simulink model "SMC_DTC_VS_DTC"  (R2023b)
settings: Solver=FixedStepAuto  StartTime=0.0  StopTime=0.8  FixedStep=0.0000001  MaxStep=0.00001  MinStep=0.0000005
libraries: spsDCVoltageSourceLib x2, spsGroundLib x2, simulink x2, spsThreePhaseVIMeasurementLib x2, spsUniversalBridgeLib x2, sps_lib x1
settings Model: SimulationMode=accelerator  Creator=rainy  LastModifiedBy=rainy
settings SolverCC: ZeroCrossAlgorithm=Adaptive
settings DebuggingCC: MaskedZcDiagnostic=none  IgnoredZcDiagnostic=none

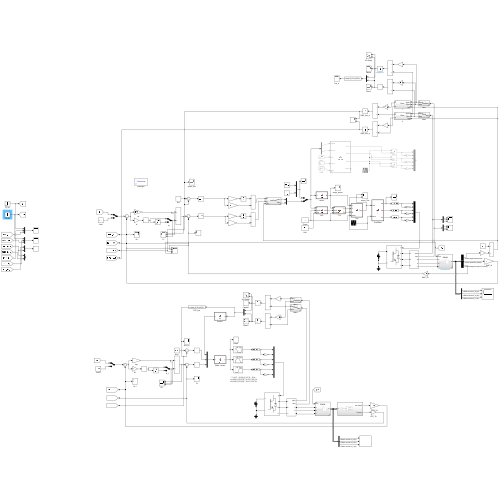
[thumbnail: Simulink's stored preview of the top-level diagram]
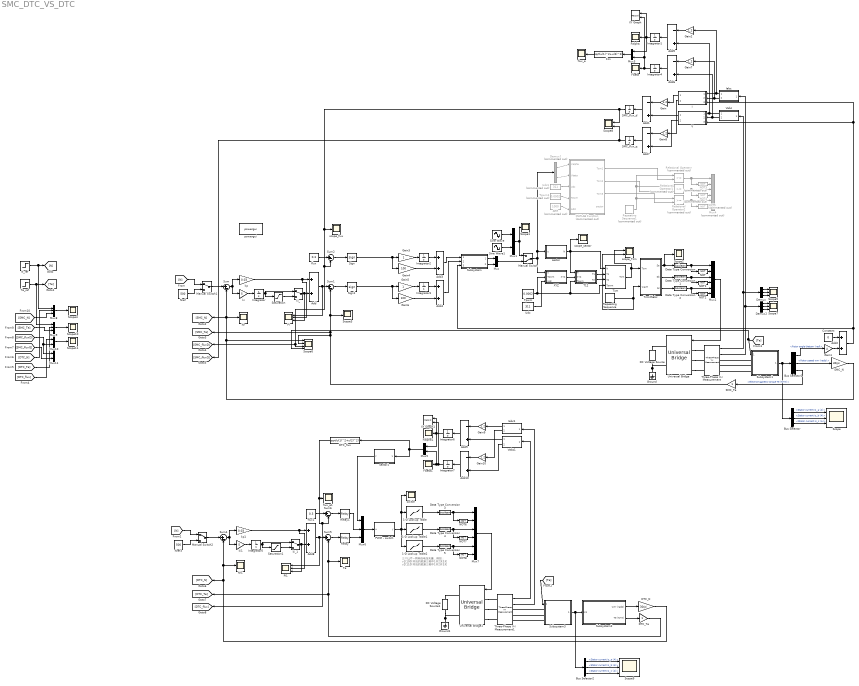
== system SMC_DTC_VS_DTC ==
  note: 三个LUT一同构成电压矢量，例如：
      | v1(100)对应的就是三相中1开2关3关
      | v2(110)对应的就是三相中1开2开3关
  1-D Lookup Table : Lookup_n-D  NumberOfTableDimensions=1  BreakpointsForDimension1=[1 2 3 4 5 6]  Table=[1 1 0 0 0 1]  InternalRulePriority=Speed  RndMeth=Simplest
  1-D Lookup Table1 : Lookup_n-D  NumberOfTableDimensions=1  BreakpointsForDimension1=[1 2 3 4 5 6]  Table=[0 1 1 1 0 0]  InternalRulePriority=Speed  RndMeth=Simplest
  1-D Lookup Table2 : Lookup_n-D  NumberOfTableDimensions=1  BreakpointsForDimension1=[1 2 3 4 5 6]  Table=[0 0 0 1 1 1]  InternalRulePriority=Speed  RndMeth=Simplest
  ARR : Constant  Commented=on  Value=1000
  Add{,2..4,8} (5 alike) : Sum
  Add{1,5..7,9..10} (6 alike) : Sum  Inputs=-+
  Bus Selector : BusSelector  OutputSignals=Stator current is_a (A),Stator current is_b (A),Stator current is_c (A)
  Bus Selector1 : BusSelector  OutputSignals=Rotor angle thetam (rad),Rotor speed wm (rad/s),Electromagnetic torque Te (N*m)
  Bus Selector2 : BusSelector  OutputSignals=Stator current is_a (A),Stator current is_b (A),Stator current is_c (A)
  Constant : Constant  Value=0
  DC Voltage Source : spsDCVoltageSourceLib/DC Voltage Source  Amplitude=311  Measurements=Voltage
  DC Voltage Source1 : spsDCVoltageSourceLib/DC Voltage Source  Amplitude=311  Measurements=Voltage
  DTC_N : Gain  Gain=30/pi
  DTC_Te : Gain
  DTC_flux : Fcn  Expr=sqrt(u(1)^2+u(2)^2)
  Data Type Conversion{,1..5} (6 alike) : DataTypeConversion  OutDataTypeStr=boolean  SaturateOnIntegerOverflow=off  RndMeth=Floor
  Demux : Demux  Outputs=3
  Demux1 : Demux  Commented=on  Outputs=2
  Demux2 : Demux  Outputs=3
  Falpha : Scope
  Falpha1 : Scope
  Fbeta : Scope
  Fbeta1 : Scope
  Fcn : Fcn  Expr=sqrt(u(1)^2+u(2)^2)
  Gain{,2,7..10} (6 alike) : Gain  Gain=1.2
  Gain1 : Gain  Gain=4
  Gain3 : Gain
  Gain4 : Gain  Gain=100
  Gain5 : Gain
  Gain6 : Gain  Gain=100
  Ground : spsGroundLib/Ground  LConnTagsString=a
  Ground1 : spsGroundLib/Ground  LConnTagsString=a
  I : Subsystem  ReferencedSubsystem=Park
  Iabc : Subsystem  ReferencedSubsystem=Clark
  Iabc1 : Subsystem  ReferencedSubsystem=Clark
  Integrator{,1..7} (8 alike) : Integrator
  MATLAB Function : MATLAB Function  Commented=on  TreatAsAtomicUnit=on
  Manual Switch : ManualSwitch  CurrentSetting=0
  Manual Switch1 : ManualSwitch
  Manual Switch2 : ManualSwitch
  Mux{,1,3,5,10..11} (6 alike) : Mux  Inputs=2
  Mux2 : Mux  Inputs=6
  Mux4 : Mux  Commented=on  Inputs=6
  Mux6 : Mux  Inputs=3
  Mux7 : Mux  Inputs=6
  Mux8 : Mux  Inputs=3
  Mux9 : Mux  Inputs=3
  NOT{,1..2,6..8} (6 alike) : Logic  Operator=NOT  IconShape=distinctive  AllPortsSameDT=off  OutDataTypeStr=boolean
  NOT3 : Logic  Commented=on  Operator=NOT  IconShape=distinctive  AllPortsSameDT=off  OutDataTypeStr=boolean
  NOT4 : Logic  Commented=on  Operator=NOT  IconShape=distinctive  AllPortsSameDT=off  OutDataTypeStr=boolean
  NOT5 : Logic  Commented=on  Operator=NOT  IconShape=distinctive  AllPortsSameDT=off  OutDataTypeStr=boolean
  N_ref : Step  Time=0.4  Before=200  After=400  SampleTime=0
  Nr : Scope
  Nr1 : Scope
  Nref : Constant  Value=500
  Nref3 : Constant  Value=500
  PI : Scope  NumInputPorts=3
  PI1 : Scope  NumInputPorts=3
  PWM - switch : MATLAB Function  TreatAsAtomicUnit=on
  Relational Operator : RelationalOperator  Commented=on  OutDataTypeStr=boolean  RndMeth=Simplest  InputSameDT=off
  Relational Operator1 : RelationalOperator  Commented=on  OutDataTypeStr=boolean  RndMeth=Simplest  InputSameDT=off
  Relational Operator2 : RelationalOperator  Commented=on  OutDataTypeStr=boolean  RndMeth=Simplest  InputSameDT=off
  Relay : Relay  OnSwitchValue=0.1  OffSwitchValue=-0.1
  Relay1 : Relay  OnSwitchValue=0.002  OffSwitchValue=-0.002
  Repeating Sequence : simulink/Sources/Repeating Sequence  rep_seq_t=[0 0.0001 0.0002]  rep_seq_y=[0 10 0]
  Repeating Sequence1 : simulink/Sources/Repeating Sequence  Commented=on  rep_seq_t=[0 0.0001 0.0002]  rep_seq_y=[0 1000 0]
  SMC_N : Gain  Gain=30/pi
  SMC_Te : Gain
  SMC_flux_d : Integrator
  SMC_flux_q : Integrator
  Saturation : Saturate  UpperLimit=10  LowerLimit=-10  ZeroCross=off
  Saturation1 : Saturate  UpperLimit=10  LowerLimit=-10
  Scope{,5,7,9} (4 alike) : Scope  NumInputPorts=3
  Scope{1..4,10..11} (6 alike) : Scope
  Scope6 : Scope  NumInputPorts=4
  Scope8 : Scope  NumInputPorts=2
  Sign : Signum
  Sign1 : Signum
  Sine Wave : Sin  Amplitude=200  Frequency=50*pi  Phase=-pi/2  SampleTime=0
  Sine Wave1 : Sin  Amplitude=200  Frequency=50*pi  SampleTime=0
  Subsystem : Subsystem  ReferencedSubsystem=AntiPark
  Subsystem1 : Subsystem  ReferencedSubsystem=PMSM
  Subsystem2 : Subsystem
  Subsystem3 : Subsystem  ReferencedSubsystem=PMSM
  Sum{,1..2,4..6} (6 alike) : Sum  Inputs=|+-
  T12 : MATLAB Function  TreatAsAtomicUnit=on
  Tcm : MATLAB Function  TreatAsAtomicUnit=on
  Tcm2Sabc : MATLAB Function  TreatAsAtomicUnit=on
  Te : Scope
  Te_ref : Step  Time=0.2  After=3  SampleTime=0
  Three-Phase V-I Measurement : spsThreePhaseVIMeasurementLib/Three-Phase V-I Measurement  VoltageMeasurement=phase-to-ground  SetLabelV=off  LabelV=Vabc  Vpu=off  VpuLL=off  CurrentMeasurement=yes  SetLabelI=off  LabelI=Iabc  Ipu=off  Pbase=100e6  Vbase=500e3  OutputType=Complex  PhasorSimulation=off  PSBequivalent=0
  Three-Phase V-I Measurement1 : spsThreePhaseVIMeasurementLib/Three-Phase V-I Measurement  VoltageMeasurement=phase-to-ground  SetLabelV=off  LabelV=Vabc  Vpu=off  VpuLL=off  CurrentMeasurement=yes  SetLabelI=off  LabelI=Iabc  Ipu=off  Pbase=100e6  Vbase=500e3  OutputType=Complex  PhasorSimulation=off  PSBequivalent=0
  Tpwm : Constant  Value=0.0002
  Tpwm1 : Constant  Commented=on  Value=0.0002
  Udc : Constant  Value=311
  Udc1 : Constant  Commented=on  Value=311
  Universal Bridge : spsUniversalBridgeLib/Universal Bridge  Arms=3  SnubberResistance=1e5  SnubberCapacitance=inf  Device=IGBT / Diodes  Ron=1e-3  Lon=0  ForwardVoltages="[  0  0  ]"  ForwardVoltage=0  GTOparameters=[ 10e-6 , 20e-6 ]  IGBTparameters=[ 1e-6 , 2e-6 ]  Measurements=None  Measurements_2=None  converterType=Rectifier
  Universal Bridge1 : spsUniversalBridgeLib/Universal Bridge  Arms=3  SnubberResistance=1e5  SnubberCapacitance=inf  Device=IGBT / Diodes  Ron=1e-3  Lon=0  ForwardVoltages="[  0  0  ]"  ForwardVoltage=0  GTOparameters=[ 10e-6 , 20e-6 ]  IGBTparameters=[ 1e-6 , 2e-6 ]  Measurements=None  Measurements_2=None  converterType=Rectifier
  V : Subsystem  ReferencedSubsystem=Park
  Vabc : Subsystem  ReferencedSubsystem=Clark
  Vabc1 : Subsystem  ReferencedSubsystem=Clark
  XY Graph : Record  FileSettingsInternal="{\"entries\":[{\"content\":{\"excelSettings\":{\"content\":{},\"type\":\"Streamout.ExcelSettings\"}},\"type\":\"Streamout.FileSettingStorage\",\"uuid\":\"\"}],\"packageUris\":[\"http:\\/\\/schema.mathworks.com\\/mf0\\/streamout_blocks\\/R2020a\"],\"version\":\"1.0\"}"  Layout=[1 1]  SignalsInternal="{\"entries\":[{\"content\":{\"signals\":[{\"content\":{\"blockPath\":[],\"dimensions\":[1],\"domain\":\"\",\"lineColor\":\"#64d413\",\"plots\":[1],\"port\":1,\"sid\":[\"\"],\"signalID\":32394,\"signalName\":\"Integrator1\"},\"type\":\"RecordBlkView.Signal\",\"uuid\":\"\"},{\"content\":{\"blockPath\":[],\"dimensions\":[1],\"domain\":\"\",\"lineColor\":\"#ff13a6\",\"plots\":[1],\"port\":2,\"sid\":[\"\"],\"signalID\":32398,\"signalName\":\"Integrator4\"},\"type\":\"RecordBlkView.Signal\",\"uuid\":\"\"}]},\"type\":\"RecordBlkView.InputSignals\",\"uuid\":\"\"}],\"packageUris\":[\"http:\\/\\/schema.mathworks.com\\/mf0\\/streamout_blocks\\/R2020a\"],\"version\":\"1.0\"}"  VisualizationBindings="{\"xyplotplugin\":{\"info\":[{\"series\":[{\"bindingParametersList\":[{\"parameter\":\"X-Axis\",\"signalID\":32394,\"signalName\":\"Integrator1\"},{\"parameter\":\"Y-Axis\",\"signalID\":32398,\"signalName\":\"Integrator4\"}],\"seriesID\":40381}],\"subplotID\":1}]}}"  CompatibilityTag=XY  st=-1
  XY Graph1 : Record  FileSettingsInternal="{\"entries\":[{\"content\":{\"excelSettings\":{\"content\":{},\"type\":\"Streamout.ExcelSettings\"}},\"type\":\"Streamout.FileSettingStorage\",\"uuid\":\"\"}],\"packageUris\":[\"http:\\/\\/schema.mathworks.com\\/mf0\\/streamout_blocks\\/R2020a\"],\"version\":\"1.0\"}"  Layout=[1 1]  SignalsInternal="{\"entries\":[{\"content\":{\"signals\":[{\"content\":{\"blockPath\":[],\"dimensions\":[1],\"domain\":\"\",\"lineColor\":\"#a2142f\",\"plots\":[1],\"port\":1,\"sid\":[\"\"],\"signalID\":32402,\"signalName\":\"Integrator6\"},\"type\":\"RecordBlkView.Signal\",\"uuid\":\"\"},{\"content\":{\"blockPath\":[],\"dimensions\":[1],\"domain\":\"\",\"lineColor\":\"#139fff\",\"plots\":[1],\"port\":2,\"sid\":[\"\"],\"signalID\":32406,\"signalName\":\"Integrator7\"},\"type\":\"RecordBlkView.Signal\",\"uuid\":\"\"}]},\"type\":\"RecordBlkView.InputSignals\",\"uuid\":\"\"}],\"packageUris\":[\"http:\\/\\/schema.mathworks.com\\/mf0\\/streamout_blocks\\/R2020a\"],\"version\":\"1.0\"}"  VisualizationBindings="{\"xyplotplugin\":{\"info\":[{\"series\":[{\"bindingParametersList\":[{\"parameter\":\"X-Axis\",\"signalID\":32402,\"signalName\":\"Integrator6\"},{\"parameter\":\"Y-Axis\",\"signalID\":32406,\"signalName\":\"Integrator7\"}],\"seriesID\":47759}],\"subplotID\":1}]}}"  CompatibilityTag=XY  st=-1
  XYZ : MATLAB Function  TreatAsAtomicUnit=on
  flux : Constant  Value=0.3
  flux1 : Constant  Value=0.3
  flux_a : Scope
  flux_a1 : Scope
  ki : Gain  Gain=5
  ki1 : Gain  Gain=5
  ki_ : ManualSwitch
  ki_1 : ManualSwitch
  kp : Gain  Gain=0.03
  kp1 : Gain  Gain=0.03
  powergui : sps_lib/powergui  Priority=1  SimulationMode=Continuous  SampleTime=50e-6  frequency=60  Iterations=50  frequencyindice=0  Pbase=100e6  ErrMax=1e-4  UnitsV=kV  UnitsW=MW  buscounter=0  FunctionMessages=off  echomessages=off  EnableUseOfTLC=off  CurrentSourceSwitches=off  DisableSnubberDevices=off  DisableRonSwitches=off  DisableVfSwitches=off  DisplayEquations=off  AutomaticDiscreteSolvers=off  SolverType=Tustin/Backward Euler (TBE)  Interpol=off  ExternalGateDelay=off  methode=off  Ts=100  x0status=blocks  SPID=on  SwTol=0  HookPort=off  NonlinearTolerance=1e-4  nMaxIteration=100  ContinueOnMaxIteration=off  RestoreLinks=warning  ResistiveCurrentMeasurement=off  Frange=[0:2:500]  Ylog=off  Xlog=on  ShowGrid=off  save=off  variable=ZData  structure=0  ZoomFFT=off  StartTime=0.0  cycles=1  DisplayStyle=1  fundamental=60  FreqAxis=off  MaxFrequency=1000  frequencyindicesteady=1  RmsSteady=1  display=off
  scope_Tcm : Scope  NumInputPorts=2
  scope_flux : Scope
  scope_sector : Scope
  sector : MATLAB Function  TreatAsAtomicUnit=on
  sector1 : MATLAB Function  TreatAsAtomicUnit=on
  switch : Scope
  wires:
  [Te] -> Scope6/4, Subsystem1/1
  Bus Selector/2 -> Scope/2  "<Stator current is_b (A)>"
  Bus Selector/3 -> Scope/3  "<Stator current is_c (A)>"
  Bus Selector/1 -> Scope/1  "<Stator current is_a (A)>"
  Bus Selector1/2 -> SMC_N/1  "<Rotor speed wm (rad/s)>"
  Bus Selector1/3 -> SMC_Te/1  "<Electromagnetic torque Te (N*m)>"
  ki_/1 -> PI/3, Add/2
  Saturation/1 -> ki_/2
  SMC_N/1 -> Scope6/1, Sum/2, [SMC_N], Nr/1
  kp/1 -> PI/2, Add/1
  Integrator/1 -> ki_/1, Saturation/1
  ki/1 -> Integrator/1
  Add/1 -> Sum1/1, PI/1
  Sum/1 -> ki/1, kp/1
  Nref/1 -> Manual Switch1/2
  Add1/1 -> SMC_flux_d/1
  Three-Phase V-I Measurement/2 -> Demux2/1, Iabc/1
  Gain/1 -> Add1/1
  Three-Phase V-I Measurement/1 -> Demux/1, Vabc/1
  Iabc/1 -> Gain2/1, I/1
  Iabc/2 -> Gain7/1, I/2
  I/1 -> Gain/1
  Vabc/1 -> Add5/2, V/1
  Vabc/2 -> V/2, Add6/2
  V/1 -> Add1/2
  flux/1 -> Sum2/1
  SMC_flux_d/1 -> Scope8/1, Scope6/3, [SMC_fluxD], Sum2/2, scope_flux/1
  Gain1/1 -> Add2/2
  Constant/1 -> Add2/1
  Bus Selector1/1 -> Gain1/1  "<Rotor angle thetam (rad)>"
  Tpwm/1 -> Tcm/4(Tpwm), T12/3(Tpwm), XYZ/2(Tpwm)
  Udc/1 -> XYZ/3(Udc)
  XYZ/1(XYZ) -> T12/2(XYZ)
  sector/1(N) -> scope_sector/1, Tcm/1(N), T12/1(N)
  T12/1(T1) -> Tcm/2(T1)
  T12/2(T2) -> Tcm/3(T2)
  Tcm/1(Tcm) -> scope_Tcm/1, Tcm2Sabc/1(Tcm)
  Repeating Sequence/1 -> Tcm2Sabc/2(wave), scope_Tcm/2
  NOT/1 -> Mux2/2
  Tcm2Sabc/3(Sc) -> Data Type Conversion2/1
  Data Type Conversion1/1 -> NOT1/1, Mux2/3
  Data Type Conversion2/1 -> NOT2/1, Mux2/5
  Tcm2Sabc/2(Sb) -> Data Type Conversion1/1
  Tcm2Sabc/1(Sa) -> Scope2/1, Data Type Conversion/1
  NOT1/1 -> Mux2/4
  Data Type Conversion/1 -> NOT/1, Mux2/1
  NOT2/1 -> Mux2/6
  Subsystem/1 -> Mux/1
  Subsystem/2 -> Mux/2
  Manual Switch/1 -> XYZ/1(u), Demux1/1, sector/1(u)
  Mux/1 -> Manual Switch/2
  Mux1/1 -> Scope1/1, Manual Switch/1
  Sine Wave/1 -> Mux1/1
  Sine Wave1/1 -> Mux1/2
  Sign/1 -> Gain4/1, Gain3/1
  Gain3/1 -> Integrator2/1
  Integrator2/1 -> Add3/1
  Gain4/1 -> Add3/2
  Sign1/1 -> Gain6/1, Gain5/1
  Gain6/1 -> Add4/2
  Integrator3/1 -> Add4/1
  Gain5/1 -> Integrator3/1
  Sum1/1 -> Sign1/1
  Sum2/1 -> Sign/1
  Add4/1 -> Subsystem/2
  Subsystem1/1 -> Bus Selector1/1, Bus Selector/1
  Demux/1 -> Scope5/1
  Demux/2 -> Scope5/2
  Demux/3 -> Scope5/3
  Demux1/1 -> MATLAB Function/1(Valpha)
  Demux1/2 -> MATLAB Function/2(Vbeta)
  Udc1/1 -> MATLAB Function/3(Udc)
  Tpwm1/1 -> MATLAB Function/4(Tpwm)
  ARR/1 -> MATLAB Function/5(ARR)
  MATLAB Function/3(Tcm3) -> Relational Operator2/2
  Relational Operator2/1 -> NOT5/1, Mux4/5
  NOT3/1 -> Mux4/2
  NOT5/1 -> Mux4/6
  Relational Operator1/1 -> NOT4/1, Mux4/3
  Relational Operator/1 -> NOT3/1, Mux4/1
  NOT4/1 -> Mux4/4
  MATLAB Function/2(Tcm2) -> Relational Operator1/2
  Repeating Sequence1/1 -> Relational Operator2/1, Relational Operator1/1, Relational Operator/1
  MATLAB Function/1(Tcm1) -> Relational Operator/2
  Mux2/1 -> Universal Bridge/1
  Add2/1 -> I/3, V/3, Subsystem/3
  Integrator1/1 -> Mux3/1, Falpha/1, XY Graph/1
  Integrator4/1 -> Mux3/2, XY Graph/2, Fbeta/1
  Gain2/1 -> Add5/1
  Add5/1 -> Integrator1/1
  Gain7/1 -> Add6/1
  Add6/1 -> Integrator4/1
  Fcn/1 -> flux_a/1
  Mux3/1 -> Fcn/1
  V/2 -> Add7/2
  Add7/1 -> SMC_flux_q/1
  I/2 -> Gain8/1
  Gain8/1 -> Add7/1
  SMC_flux_q/1 -> [SMC_fluxQ], Scope8/2
  Demux2/3 -> Scope7/3
  Demux2/2 -> Scope7/2
  Demux2/1 -> Scope7/1
  Add3/1 -> Subsystem/1
  Manual Switch1/1 -> Sum/1
  [N] -> Manual Switch1/1
  Integrator7/1 -> XY Graph1/2, Mux5/2, Fbeta1/1
  Add8/1 -> PI1/1, Sum5/1
  Data Type Conversion4/1 -> Mux7/3, NOT7/1
  Iabc1/2 -> Gain10/1
  Mux5/1 -> sector1/1(u), DTC_flux/1
  Add10/1 -> Integrator7/1
  Vabc1/2 -> Add10/2
  Integrator6/1 -> XY Graph1/1, Mux5/1, Falpha1/1
  Bus Selector2/2 -> Scope9/2  "<Stator current is_b (A)>"
  Relay/1 -> Mux6/3
  NOT7/1 -> Mux7/4
  Three-Phase V-I Measurement1/2 -> Iabc1/1
  Subsystem3/1 -> Bus Selector2/1, Subsystem2/1(In1)
  ki_1/1 -> PI1/3, Add8/2
  1-D Lookup Table1/1 -> Data Type Conversion4/1
  NOT6/1 -> Mux7/2
  Integrator5/1 -> ki_1/1, Saturation1/1
  sector1/1(y) -> Mux6/1
  Relay1/1 -> Mux6/2
  Mux7/1 -> Universal Bridge1/1
  1-D Lookup Table2/1 -> Data Type Conversion5/1
  PWM - switch/1(y) -> 1-D Lookup Table2/1, switch/1, 1-D Lookup Table/1, 1-D Lookup Table1/1
  Saturation1/1 -> ki_1/2
  1-D Lookup Table/1 -> Data Type Conversion3/1
  Manual Switch2/1 -> Sum4/1
  Data Type Conversion3/1 -> NOT6/1, Mux7/1
  Gain10/1 -> Add10/1
  Mux6/1 -> PWM - switch/1(u)
  Bus Selector2/1 -> Scope9/1  "<Stator current is_a (A)>"
  DTC_flux/1 -> Sum6/2, [DTC_flux], flux_a1/1
  Sum5/1 -> Relay/1
  Vabc1/1 -> Add9/2
  Data Type Conversion5/1 -> Mux7/5, NOT8/1
  Subsystem2/2(Te (N*m)) -> DTC_Te/1
  DTC_N/1 -> [DTC_N], Sum4/2, Nr1/1
  Subsystem2/1(wm (rad/s)) -> DTC_N/1
  kp1/1 -> PI1/2, Add8/1
  Add9/1 -> Integrator6/1
  Bus Selector2/3 -> Scope9/3  "<Stator current is_c (A)>"
  Iabc1/1 -> Gain9/1
  Sum6/1 -> Relay1/1
  Sum4/1 -> ki1/1, kp1/1
  flux1/1 -> Sum6/1
  Gain9/1 -> Add9/1
  Three-Phase V-I Measurement1/1 -> Vabc1/1
  ki1/1 -> Integrator5/1
  NOT8/1 -> Mux7/6
  N_ref/1 -> Mux8/1, [N]
  [N] -> Manual Switch2/1
  Nref3/1 -> Manual Switch2/2
  [Te] -> Subsystem3/1
  Te_ref/1 -> Mux9/1, [Te]
  DTC_Te/1 -> [DTC_Te], Te/1, Sum5/2
  SMC_Te/1 -> [SMC_Te], Sum1/2, Scope3/1, Scope6/2
  [SMC_N] -> Mux8/3
  [DTC_N] -> Mux8/2
  [SMC_Te] -> Mux9/3
  [DTC_Te] -> Mux9/2
  [SMC_fluxD] -> Mux10/2, Mux11/1
  [DTC_flux] -> Mux10/1
  [SMC_fluxQ] -> Mux11/2
  Mux8/1 -> Scope4/1
  Mux9/1 -> Scope10/1
  Mux10/1 -> Scope11/1
  connections:
  Ground/LConn1 -- Universal Bridge/RConn2 -- DC Voltage Source/LConn1
  Universal Bridge/LConn3 -- Three-Phase V-I Measurement/LConn3
  Subsystem1/LConn3 -- Three-Phase V-I Measurement/RConn3
  Subsystem1/LConn1 -- Three-Phase V-I Measurement/RConn1
  Universal Bridge/LConn2 -- Three-Phase V-I Measurement/LConn2
  Subsystem1/LConn2 -- Three-Phase V-I Measurement/RConn2
  Universal Bridge/LConn1 -- Three-Phase V-I Measurement/LConn1
  DC Voltage Source/RConn1 -- Universal Bridge/RConn1
  Ground1/LConn1 -- Universal Bridge1/RConn2 -- DC Voltage Source1/LConn1
  Subsystem3/LConn3 -- Three-Phase V-I Measurement1/RConn3
  Subsystem3/LConn1 -- Three-Phase V-I Measurement1/RConn1
  Subsystem3/LConn2 -- Three-Phase V-I Measurement1/RConn2
  Universal Bridge1/LConn2 -- Three-Phase V-I Measurement1/LConn2
  Universal Bridge1/LConn1 -- Three-Phase V-I Measurement1/LConn1
  Universal Bridge1/LConn3 -- Three-Phase V-I Measurement1/LConn3
  DC Voltage Source1/RConn1 -- Universal Bridge1/RConn1

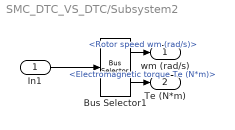
== system SMC_DTC_VS_DTC/Subsystem2 ==
  In1 : Inport
  Bus Selector1 : BusSelector  OutputSignals=Rotor speed wm (rad/s),Electromagnetic torque Te (N*m)
  wm (rad/s) : Outport
  Te (N*m) : Outport  Port=2
  wires:
  Bus Selector1/2 -> Te (N*m)/1  "<Electromagnetic torque Te (N*m)>"
  Bus Selector1/1 -> wm (rad/s)/1  "<Rotor speed wm (rad/s)>"
  In1/1 -> Bus Selector1/1

== matlab function SMC_DTC_VS_DTC/XYZ ==
  data: u input; XYZ output; Tpwm input; Udc input
function XYZ = fcn(u, Tpwm, Udc)

XYZ = zeros([1 3]);
XYZ(1) = Tpwm/Udc * sqrt(3)*u(2);
XYZ(2) = Tpwm/Udc * (3/2*u(1) + sqrt(3)/2*u(2));
XYZ(3) = Tpwm/Udc * (-3/2*u(1) + sqrt(3)/2*u(2));

== matlab function SMC_DTC_VS_DTC/sector ==
  data: u input; N output
function N = fcn(u)

if(u(1) == 0)
    i = 4;
else
    % 将\psi_{\aplha}和\psi_{\beta}分解为三相
    a1 = u(2);
    b1 = u(2)*(-0.5) + sqrt(3)/2*u(1);
    c1 = u(2)*(-0.5) - sqrt(3)/2*u(1);

    if(a1 > 0)
        a = 1;
    else
        a = 0;
    end
    
    if(b1 > 0)
        b = 1;
    else
        b = 0;
    end
    
    if(c1 > 0)
        c = 1;
    else
        c = 0;
    end

    % i = 4*a+2*b+c;
    i = 4*c+2*b+a;
end

% Sector_table=[4 6 5 2 3 1];
% 
% N = Sector_table(i);
N = i;

== matlab function SMC_DTC_VS_DTC/T12 ==
  data: N input; XYZ input; T1 output; Tpwm input; T2 output
function [T1, T2] = fcn(N, XYZ, Tpwm)

X = XYZ(1);
Y = XYZ(2);
Z = XYZ(3);

switch (N)
    case 1
        T1 = Z; T2 = Y;
    case 2
        T1 = Y; T2 = -X;
    case 3
        T1 = -Z; T2 = X;
    case 4
        T1 = -X; T2 = Z;
    case 5
        T1 = X; T2 = -Y;
    otherwise
        T1 = -Y; T2 = -Z;
end

if T1 + T2 > Tpwm
    T1 = T1/(T1 + T2)*Tpwm;
    T2 = T2/(T1 + T2)*Tpwm;
end

== matlab function SMC_DTC_VS_DTC/Tcm ==
  data: N input; T1 input; T2 input; Tcm output; Tpwm input
function Tcm = fcn(N, T1, T2, Tpwm)

Tcm = zeros([1 3]);

Ta = (Tpwm - T1 - T2)/4;
Tb = Ta + T1/2;
Tc = Tb + T2/2;

switch(N)
    case 1
        Tcm(1) = Tb;
        Tcm(2) = Ta;
        Tcm(3) = Tc;
    case 2
        Tcm(1) = Ta;
        Tcm(2) = Tc;
        Tcm(3) = Tb;
    case 3
        Tcm(1) = Ta;
        Tcm(2) = Tb;
        Tcm(3) = Tc;
    case 4
        Tcm(1) = Tc;
        Tcm(2) = Tb;
        Tcm(3) = Ta;
    case 5
        Tcm(1) = Tc;
        Tcm(2) = Ta;
        Tcm(3) = Tb;
    otherwise
        Tcm(1) = Tb;
        Tcm(2) = Tc;
        Tcm(3) = Ta;
end

Tcm = Tcm * 100000;

== matlab function SMC_DTC_VS_DTC/Tcm2Sabc ==
  data: Tcm input; wave input; Sa output; Sb output; Sc output
function [Sa, Sb, Sc]= fcn(Tcm, wave)

if(wave - Tcm(1) > 0)
    Sa = 1;
else
    Sa = 0;
end

if(wave - Tcm(2) > 0)
    Sb = 1;
else
    Sb = 0;
end

if(wave - Tcm(3) > 0)
    Sc = 1;
else
    Sc = 0;
end

== matlab function SMC_DTC_VS_DTC/MATLAB Function ==
  data: Valpha input; Tcm1 output; Vbeta input; Udc input; Tpwm input; ARR input; Tcm2 output; Tcm3 output; sector output
function [Tcm1,Tcm2,Tcm3,sector] = SVPWM(Valpha,Vbeta,Udc,Tpwm,ARR)

%输出变量初始化
Tcm1 = 0;
Tcm2 = 0;
Tcm3 = 0;
sector = 0;


%扇区计算
%N与扇区对应的关系
%  3   1   5    4  6  2
%  I  II  III  IV  V  VI

Vref1 = Vbeta;
Vref2 = (sqrt(3)*Valpha-Vbeta)/2;
Vref3 = (-sqrt(3)*Valpha-Vbeta)/2;

if(Vref1>0)
    sector = 1;
end

if(Vref2>0)
    sector = sector+2;
end

if(Vref3>0)
    sector = sector+4;
end


%扇区内合成矢量作用时间计算
X = sqrt(3)*Vbeta*Tpwm/Udc;
Y = Tpwm/Udc*(3/2*Valpha+sqrt(3)/2*Vbeta);
Z = Tpwm/Udc*(-3/2*Valpha+sqrt(3)/2*Vbeta);

switch(sector)
    case 1
        T1 = Z;T2 = Y;
    case 2
        T1 = Y;T2 = -X;
    case 3
        T1 = -Z;T2 = X;
    case 4
        T1 = -X;T2 = Z;
    case 5
        T1 = X;T2 = -Y;
    otherwise
        T1 = -Y;T2 = -Z;
end

%过调制处理
if(T1+T2>Tpwm)
    T1 = Tpwm*T1/(T1+T2);
    T2 = Tpwm*T2/(T1+T2);
else
    T1 = T1;
    T2 = T2;
end


%扇区内合成矢量切换点时间计算
%此处为7段式，两个零矢量000 111 111插在中间，000均分插在两端
ta = (Tpwm-(T1+T2))/4;
tb = ta+T1/2;
tc = tb+T2/2;


%输出调制信号
switch(sector)
    case 1
        Tcm1 = tb;
        Tcm2 = ta;
        Tcm3 = tc;
    case 2
        Tcm1 = ta;
        Tcm2 = tc;
        Tcm3 = tb;
    case 3
        Tcm1 = ta;
        Tcm2 = tb;
        Tcm3 = tc;
    case 4
        Tcm1 = tc;
        Tcm2 = tb;
        Tcm3 = ta;
    case 5
        Tcm1 = tc;
        Tcm2 = ta;
        Tcm3 = tb;
    case 6
        Tcm1 = tb;
        Tcm2 = tc;
        Tcm3 = ta;
end


%调制信号处理，生成输入到MCU中的调制信号
Tcm1 = 2*Tcm1/Tpwm; 
Tcm2 = 2*Tcm2/Tpwm;
Tcm3 = 2*Tcm3/Tpwm;

Tcm1 = Tcm1*ARR; 
Tcm2 = Tcm2*ARR; 
Tcm3 = Tcm3*ARR;

end

== matlab function SMC_DTC_VS_DTC/PWM - switch ==
  data: u input; y output
function y = fcn(u)

% u(1) 扇区
% u(2) 磁链
% u(3) 转矩

V_Table=[5 6 1 2 3 4;3 4 5 6 1 2;6 1 2 3 4 5;2 3 4 5 6 1];
x=2*u(2)+u(3)+1;

y = V_Table(x, u(1));

== matlab function SMC_DTC_VS_DTC/sector1 ==
  data: u input; y output
function y = fcn(u)

if(u(2) == 0)
    N = 3;
else
    % 将\psi_{\aplha}和\psi_{\beta}分解为三相
    a1 = u(1);
    b1 = u(1)*(-0.5) + sqrt(3)/2*u(2);
    c1 = u(1)*(-0.5) - sqrt(3)/2*u(2);
    
    % a1 > 0，有扇区126
    % b1 > 0，有扇区234
    % c1 > 0，有扇区456
    % n为a1 b1 c1中>0的个数，0 < n < 3
    % 
    % a b c | s
    %-------|---
    % 0 0 1 | 2
    % 0 1 0 | 6
    % 0 1 1 | 1
    % 1 0 0 | 4
    % 1 0 1 | 3
    % 1 1 0 | 5

    if(a1 > 0)
        a = 0;
    else
        a = 1;
    end
    
    if(b1 > 0)
        b = 0;
    else
        b = 1;
    end
    
    if(c1 > 0)
        c = 0;
    else
        c = 1;
    end

    N = 4*a+2*b+c;
end

Sector_table=[2 6 1 4 3 5];

y = Sector_table(N);
